simulink model "untitled"  (R2018a)
settings: Solver=VariableStepAuto  StartTime=0.0  StopTime=2000.0  RelTol=1e-3
settings Model: Creator=Dani  LastModifiedBy=Dani

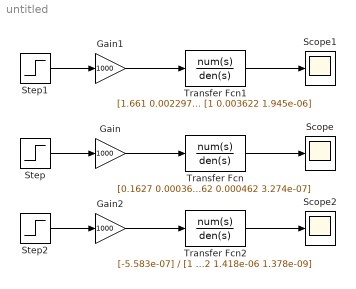
== system untitled ==
  Gain : Gain  Gain=1000
  Gain1 : Gain  Gain=1000
  Gain2 : Gain  Gain=1000
  Scope : Scope
  Scope1 : Scope
  Scope2 : Scope
  Step : Step  Time=468  Before=1  After=0  SampleTime=1
  Step1 : Step  Time=468  Before=1  After=0  SampleTime=1
  Step2 : Step  Time=468  Before=1  After=0  SampleTime=1
  Transfer Fcn : TransferFcn  Numerator=[0.1627 0.0003648]  Denominator=[1 0.09562 0.000462 3.274e-07]
  Transfer Fcn1 : TransferFcn  Numerator=[1.661 0.002297]  Denominator=[1 0.003622 1.945e-06]
  Transfer Fcn2 : TransferFcn  Numerator=[-5.583e-07]  Denominator=[1 0.01821 0.0002922 1.418e-06 1.378e-09]
  wires:
  Gain/1 -> Transfer Fcn/1
  Transfer Fcn/1 -> Scope/1
  Step/1 -> Gain/1
  Gain1/1 -> Transfer Fcn1/1
  Transfer Fcn1/1 -> Scope1/1
  Step1/1 -> Gain1/1
  Step2/1 -> Gain2/1
  Transfer Fcn2/1 -> Scope2/1
  Gain2/1 -> Transfer Fcn2/1
